simulink model "hw3_simulink"  (R2021a)
settings: Solver=VariableStepAuto  StartTime=0.0  StopTime=10.0  RelTol=1e-3
values from neighbouring files (symbols this model uses):
  A = [-2 19 20 ... (first row only)    [homework3.m]
  B = [1 ... (first row only)    [homework3.m]
  C = [0 0 3]    [homework3.m]
  F = -[1 0 0]*(Am - A)    [homework3.m]
settings Model: Creator=becke  LastModifiedBy=becke

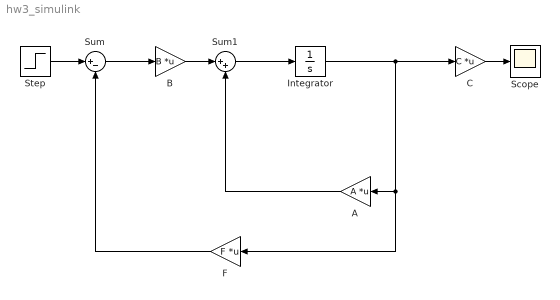
== system hw3_simulink ==
  A : Gain  Gain=A  Multiplication=Matrix(K*u)
  B : Gain  Gain=B  Multiplication=Matrix(K*u)
  C : Gain  Gain=C  Multiplication=Matrix(K*u)
  F : Gain  Gain=F  Multiplication=Matrix(K*u)
  Integrator : Integrator
  Scope : Scope
  Step : Step  SampleTime=0
  Sum : Sum  Inputs=|+-
  Sum1 : Sum  Inputs=|++
  wires:
  A/1 -> Sum1/2
  Step/1 -> Sum/1
  Sum/1 -> B/1
  B/1 -> Sum1/1
  Sum1/1 -> Integrator/1
  C/1 -> Scope/1
  Integrator/1 -> F/1, A/1, C/1
  F/1 -> Sum/2
